simulink model "Model"  (R2022b)
settings: Solver=ode4  StartTime=0.0  StopTime=0.005  FixedStep=0.000001  RelTol=1e-3
values from neighbouring files (symbols this model uses):
  C1 = 1E-6    (= 1e-06)    [para.m]
  C2 = 330E-6    (= 0.00033)    [para.m]
  L = 1E-3    (= 0.001)    [para.m]
  R1 = 100e-3    (= 0.1)    [para.m]
  R2 = 3.4    [para.m]
settings Model: Creator=nkrouglicof  LastModifiedBy=damie
settings ModelReferenceCC: EnableRefExpFcnMdlSchedulingChecks=on

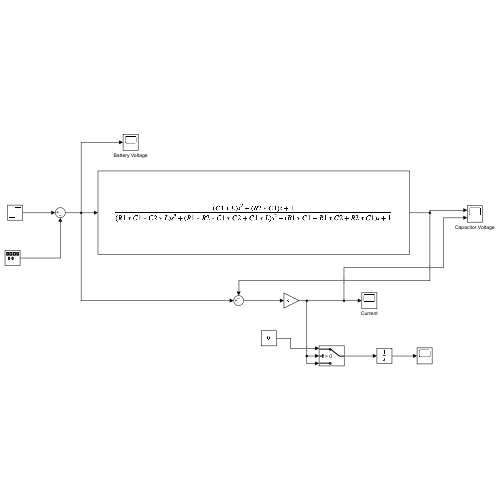
[thumbnail: Simulink's stored preview of the top-level diagram]
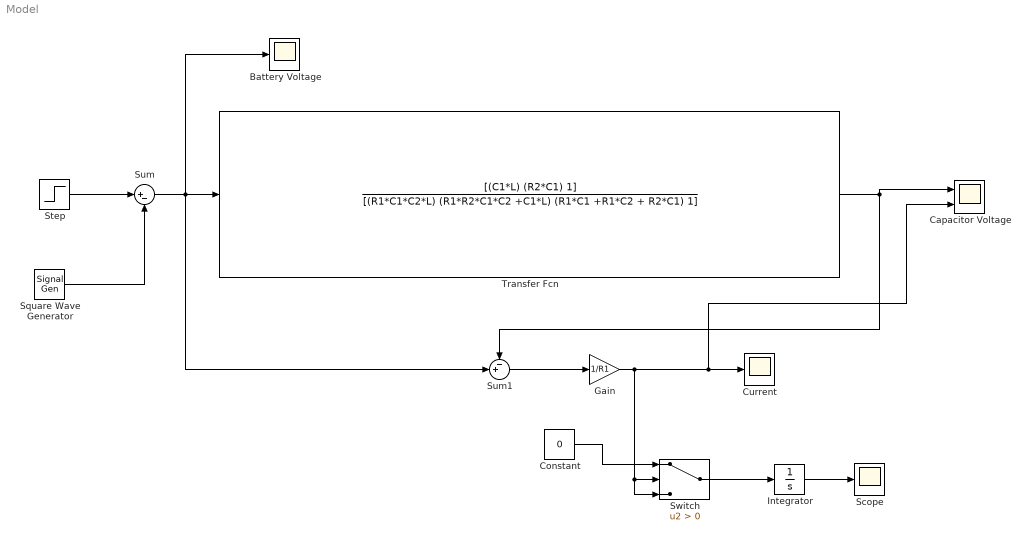
== system Model ==
  Battery Voltage : Scope
  Capacitor Voltage : Scope  NumInputPorts=2
  Constant : Constant  Value=0
  Current : Scope
  Gain : Gain  Gain=1/R1
  Integrator : Integrator
  Scope : Scope
  Square Wave Generator : SignalGenerator  WaveForm=square  Amplitude=0.1  Frequency=3000  Units=rad/sec
  Step : Step  Time=0  After=4  SampleTime=0
  Sum : Sum  Inputs=|+-
  Sum1 : Sum  Inputs=-+|
  Switch : Switch  Criteria=u2 > Threshold  SaturateOnIntegerOverflow=off  InputSameDT=off
  Transfer Fcn : TransferFcn  Numerator=[(C1*L) (R2*C1) 1]  Denominator=[(R1*C1*C2*L) (R1*R2*C1*C2 +C1*L) (R1*C1 +R1*C2 + R2*C1) 1]
  wires:
  Transfer Fcn/1 -> Sum1/1, Capacitor Voltage/1
  Step/1 -> Sum/1
  Square Wave Generator/1 -> Sum/2
  Sum/1 -> Battery Voltage/1, Sum1/2, Transfer Fcn/1
  Sum1/1 -> Gain/1
  Constant/1 -> Switch/1
  Gain/1 -> Switch/3, Switch/2, Capacitor Voltage/2, Current/1
  Switch/1 -> Integrator/1
  Integrator/1 -> Scope/1
